simulink model "System"  (R2017b)
settings: Solver=VariableStepAuto  StartTime=0.0  StopTime=8000  RelTol=1e-3
settings Model: Creator=Kim  LastModifiedBy=Kim

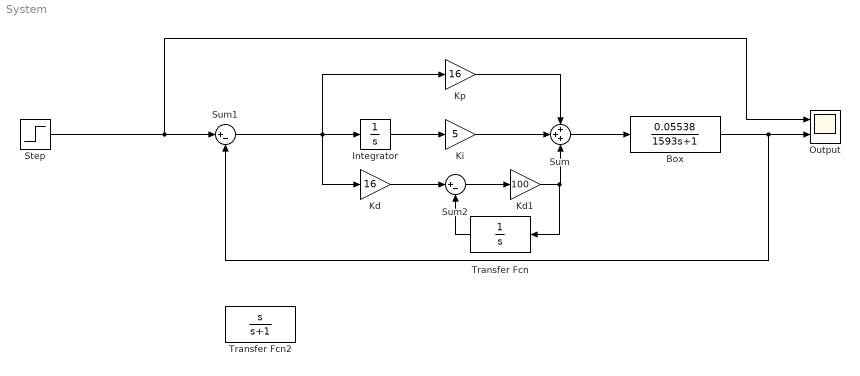
== system System ==
  Box : TransferFcn  Numerator=[0.05538]  Denominator=[1593 1]
  Integrator : Integrator
  Kd : Gain  Gain=16
  Kd1 : Gain  Gain=100
  Ki : Gain  Gain=5
  Kp : Gain  Gain=16
  Output : Scope  NumInputPorts=2
  Step : Step  After=10  SampleTime=0
  Sum : Sum  Inputs=+++
  Sum1 : Sum  Inputs=|+-
  Sum2 : Sum  Inputs=|+-
  Transfer Fcn : TransferFcn  Denominator=[1 0]
  Transfer Fcn2 : TransferFcn  Numerator=[1 0]  Denominator=[1 1]
  wires:
  Integrator/1 -> Ki/1
  Kp/1 -> Sum/1
  Box/1 -> Sum1/2, Output/2
  Sum1/1 -> Kd/1, Kp/1, Integrator/1
  Ki/1 -> Sum/2
  Sum/1 -> Box/1
  Step/1 -> Output/1, Sum1/1
  Kd/1 -> Sum2/1
  Sum2/1 -> Kd1/1
  Kd1/1 -> Transfer Fcn/1, Sum/3
  Transfer Fcn/1 -> Sum2/2
